simulink library "DYN_TIME"  (Simulink 8.8)
settings: Solver=ode45  StartTime=0.0  StopTime=10.0  RelTol=1e-3  EnableMultiTasking=on
undefined symbols (not defined in the file): DYN_par
libraries: LIB_TIME x1
settings Model: Creator=alger  LastModifiedBy=alger

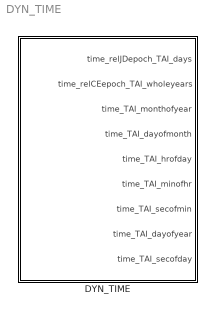
== system DYN_TIME ==
  DYN_TIME : Subsystem

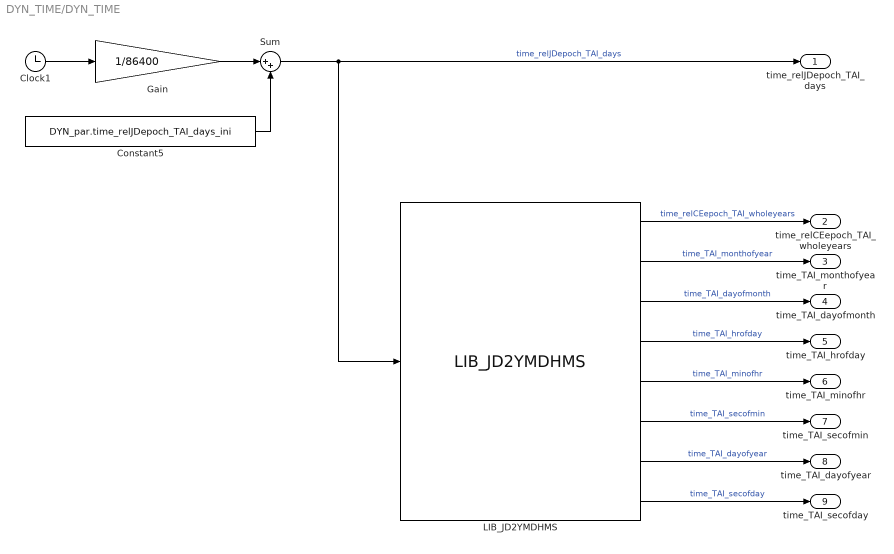
== system DYN_TIME/DYN_TIME ==
  Clock1 : Clock
  Constant5 : Constant  Value=DYN_par.time_relJDepoch_TAI_days_ini
  Gain : Gain  Gain=1/86400
  LIB_JD2YMDHMS : LIB_TIME/LIB_JD2YMDHMS
  Sum : Sum  Inputs=|++
  time_relJDepoch_TAI_days : Outport
  time_relCEepoch_TAI_wholeyears : Outport  Port=2
  time_TAI_monthofyear : Outport  Port=3
  time_TAI_dayofmonth : Outport  Port=4
  time_TAI_hrofday : Outport  Port=5
  time_TAI_minofhr : Outport  Port=6
  time_TAI_secofmin : Outport  Port=7
  time_TAI_dayofyear : Outport  Port=8
  time_TAI_secofday : Outport  Port=9
  wires:
  Constant5/1 -> Sum/2
  Clock1/1 -> Gain/1
  Gain/1 -> Sum/1
  Sum/1 -> LIB_JD2YMDHMS/1, time_relJDepoch_TAI_days/1  "time_relJDepoch_TAI_days"
  LIB_JD2YMDHMS/2 -> time_TAI_monthofyear/1  "time_TAI_monthofyear"
  LIB_JD2YMDHMS/1 -> time_relCEepoch_TAI_wholeyears/1  "time_relCEepoch_TAI_wholeyears"
  LIB_JD2YMDHMS/3 -> time_TAI_dayofmonth/1  "time_TAI_dayofmonth"
  LIB_JD2YMDHMS/4 -> time_TAI_hrofday/1  "time_TAI_hrofday"
  LIB_JD2YMDHMS/5 -> time_TAI_minofhr/1  "time_TAI_minofhr"
  LIB_JD2YMDHMS/6 -> time_TAI_secofmin/1  "time_TAI_secofmin"
  LIB_JD2YMDHMS/7 -> time_TAI_dayofyear/1  "time_TAI_dayofyear"
  LIB_JD2YMDHMS/8 -> time_TAI_secofday/1  "time_TAI_secofday"
